simulink model "BF_sans_controleur"  (R2021b)
settings: Solver=VariableStepAuto  StartTime=0.0  StopTime=10.0  RelTol=1e-3
values from neighbouring files (symbols this model uses):
  A = [0 0 0  1 0 0   0 0 0   0 0 0 ... (first row only)    [systune_gain_scheduling.m]    (also in systune_variable_gain_scheduling_LPV.m)
  B = [0 0 0 0 ... (first row only)    [systune_gain_scheduling.m]    (also in systune_variable_gain_scheduling_LPV.m)
  B2 = [0 0 ... (first row only)    [systune_gain_scheduling.m]    (also in systune_variable_gain_scheduling_LPV.m)
  C = eye(12)    [systune_gain_scheduling.m]    (also in systune_variable_gain_scheduling_LPV.m)
  C_control = [1 0 0 0 0 0 0 0 0 1 0 0 ... (96 elements, 8x12)]    [matrix_systune.mat]    (also in systune_gain_scheduling.m = [C(1:7,:);C(9,:)]; systune_variable_gain_scheduling_LPV.m = [C(1:7,:);C(9:12,:)])
  D = zeros(12,6)    [systune_gain_scheduling.m]    (also in systune_variable_gain_scheduling_LPV.m)
  x_12 = [[0; 0; 0]; [0; 0; 0]; [0; sin(angle/2); 0]; [0; 0; 0]]    [systune_gain_scheduling.m]    (also in systune_variable_gain_scheduling_LPV.m)
settings Model: Creator=florian  LastModifiedBy=florian

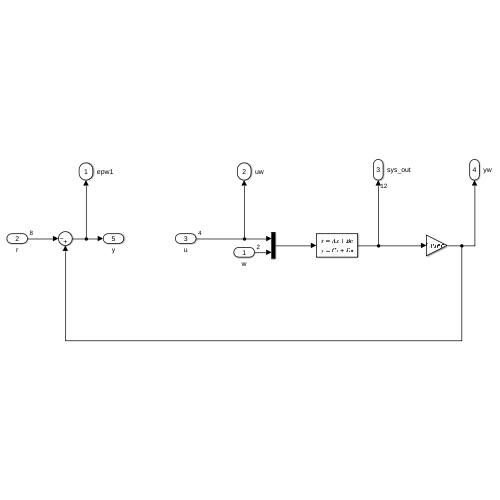
[thumbnail: Simulink's stored preview of the top-level diagram]
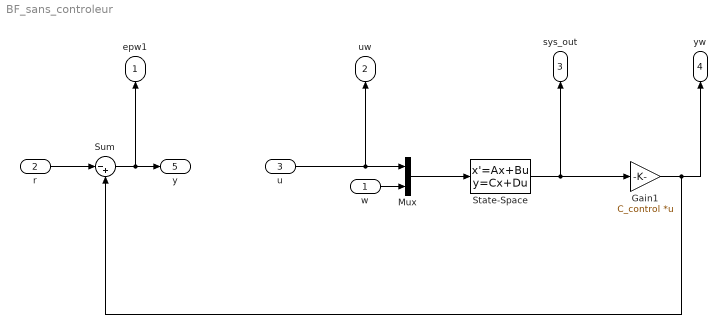
== system BF_sans_controleur ==
  w : Inport  PortDimensions=2
  r : Inport  Port=2  PortDimensions=8
  u : Inport  Port=3  PortDimensions=4
  Gain1 : Gain  Gain=C_control  Multiplication=Matrix(K*u) (u vector)
  Mux : Mux  Inputs=2
  State-Space : StateSpace  A=A  B=[B, B2]  C=C  D=D  InitialCondition=x_12
  Sum : Sum  Inputs=|-+
  epw1 : Outport  InitialOutput=0
  uw : Outport  Port=2  InitialOutput=0
  sys_out : Outport  Port=3  PortDimensions=12
  yw : Outport  Port=4
  y : Outport  Port=5
  wires:
  Mux/1 -> State-Space/1
  w/1 -> Mux/2
  r/1 -> Sum/1
  Sum/1 -> epw1/1, y/1
  State-Space/1 -> Gain1/1, sys_out/1
  Gain1/1 -> yw/1, Sum/2
  u/1 -> uw/1, Mux/1
